simulink model "ElectricalThermalSystem"  (R2026b)
settings: Solver=VariableStepAuto
undefined symbols (not defined in the file): CtrlThrBattTrgTemp, CtrlThrCabTrgTemp, CtrlThrDCDCTrgTemp, CtrlThrEMTrgTemp, CtrlThrIceTrgTemp, CtrlThrMinSpd, CtrlThrTmDelay, EnvAirTemp, PlntBattCp, PlntBattMass, PlntDCDCMass, PlntEMCp, PlntEMMass, PlntEngFuelLhv, PlntThrAirCp, PlntThrAirCpBpt, PlntThrBattTau, PlntThrCabHtc, PlntThrCabNPass, PlntThrCabTau, PlntThrCabVolume, PlntThrCoolCp, PlntThrCoolCpBpt, PlntThrCOPc, PlntThrCOPe, PlntThrDCDCTau, PlntThrDoorsArea, PlntThrDoorsK, PlntThrDoorsTk, PlntThrEMTau, PlntThrGlassArea, PlntThrGlassK, PlntThrGlassTk, PlntThrICETau, PlntThrRoofArea, PlntThrRoofK, PlntThrRoofTk
libraries: simulink x2, autolibutils x1
settings Model: ModifiedByFormat=The MathWorks, Inc.  Creator=The MathWorks, Inc.  LastModifiedBy=The MathWorks, Inc.
settings RTWCC: LargeConstantGeneration=WriteOnlyDNNConstantsToDataFiles

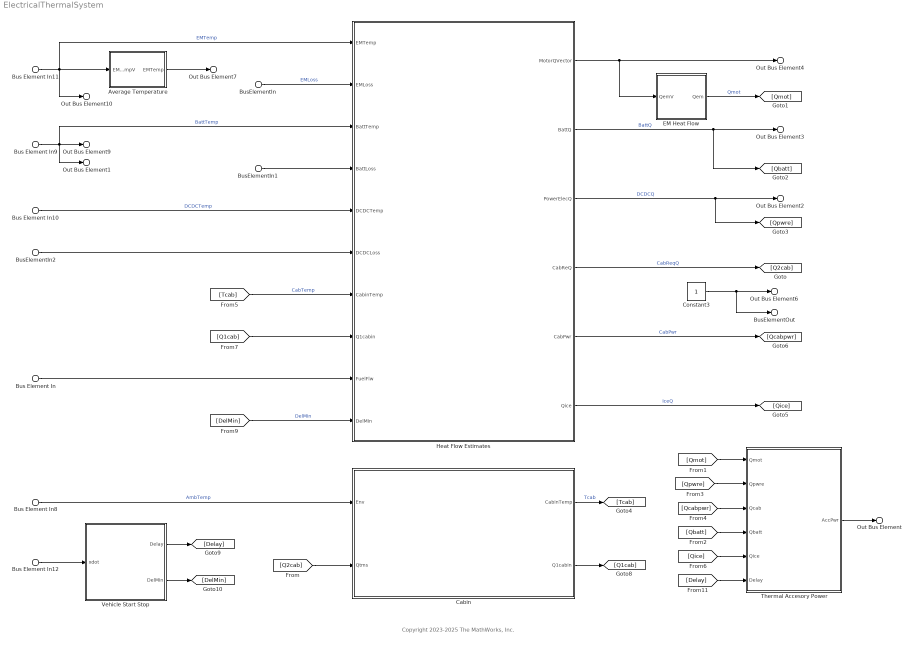
== system ElectricalThermalSystem ==
  note: Copyright 2023-2025 The MathWorks, Inc.
  Bus Element In8 : Inport  PortName=Env  Element=AmbTemp
  Bus Element In9 : Inport  Port=2  PortName=Battery  Element=BattInfo.BattTemp
  BusElementIn1 : Inport  Port=2  PortName=Battery  Element=BattInfo.BattPwrLoss
  Bus Element In10 : Inport  Port=3  PortName=PwrElec  Element=PwrETemp
  BusElementIn2 : Inport  Port=3  PortName=PwrElec  Element=PwrELoss
  Bus Element In11 : Inport  Port=4  PortName=ElecMachine  Element=EMTemp
  BusElementIn : Inport  Port=4  PortName=ElecMachine  Element=EMPwrLoss
  Bus Element In12 : Inport  Port=5  PortName=VehBody  Element=BdyFrm.Cg.Vel.xdot
  Bus Element In : Inport  Port=6  PortName=Eng  Element=FuelFlw
  Average Temperature : Subsystem
  Cabin : Subsystem
  Constant3 : Constant  SampleTime=-1
  EM Heat Flow : Subsystem  Variant=on
  Heat Flow Estimates : Subsystem
  Thermal Accesory Power : Subsystem  mask{COPe=PlntThrCOPe, COPc=PlntThrCOPc}
      mask prompts: COPe "E-Cab coefficient of performance, COPe []"; COPc "ICE coefficient of performance, COPc []"
      mask help: Estimates the power required to operate the thermal management. E-Cab coefficient of performance is the ratio of the absolute value of heat transferred to or from all electric subsystems and cabin over the power required. ICE coefficient of performance is the ratio of heat transferred to cool the internal combustion engine over the power required (applies only to HEV).
  Vehicle Start Stop : Subsystem
  Out Bus Element7 : Outport  PortName=Thermal  Element=EMCoolTempOut
  Out Bus Element9 : Outport  PortName=Thermal  Element=BattTemp
  Out Bus Element10 : Outport  PortName=Thermal  Element=MotorTemp
  Out Bus Element6 : Outport  PortName=Thermal  Element=CondPress
  Out Bus Element : Outport  PortName=Thermal  Element=EAccPwr
  Out Bus Element1 : Outport  PortName=Thermal  Element=BattCoolTemp
  Out Bus Element3 : Outport  PortName=Thermal  Element=Qbatt
  Out Bus Element2 : Outport  PortName=Thermal  Element=Qpwre
  Out Bus Element4 : Outport  PortName=Thermal  Element=Qem
  BusElementOut : Outport  PortName=Thermal  Element=EvapPress
  wires:
  Bus Element In/1 -> Heat Flow Estimates/9(FuelFlw)
  [Delay] -> Thermal Accesory Power/6(Delay)
  Bus Element In12/1 -> Vehicle Start Stop/1(xdot)
  Vehicle Start Stop/2(DelMin) -> [DelMin]
  Vehicle Start Stop/1(Delay) -> [Delay]
  Heat Flow Estimates/5(CabPwr) -> [Qcabpwr]  "CabPwr"
  Heat Flow Estimates/6(Qice) -> [Qice]  "IceQ"
  [Tcab] -> Heat Flow Estimates/7(CabinTemp)  "CabTemp"
  Cabin/1(CabinTemp) -> [Tcab]  "Tcab"
  Thermal Accesory Power/1(AccPwr) -> Out Bus Element/1
  [Qbatt] -> Thermal Accesory Power/4(Qbatt)
  [Qcabpwr] -> Thermal Accesory Power/3(Qcab)
  [Qpwre] -> Thermal Accesory Power/2(Qpwre)
  [Qmot] -> Thermal Accesory Power/1(Qmot)
  Bus Element In10/1 -> Heat Flow Estimates/5(DCDCTemp)  "DCDCTemp"
  Heat Flow Estimates/2(BattQ) -> [Qbatt], Out Bus Element3/1  "BattQ"
  Heat Flow Estimates/1(MotorQVector) -> Out Bus Element4/1, EM Heat Flow/1(QemV)
  EM Heat Flow/1(Qem) -> [Qmot]  "Qmot"
  Bus Element In8/1 -> Cabin/1(Env)  "AmbTemp"
  Constant3/1 -> Out Bus Element6/1, BusElementOut/1
  [Q2cab] -> Cabin/2(Qtms)
  Bus Element In9/1 -> Heat Flow Estimates/3(BattTemp), Out Bus Element1/1, Out Bus Element9/1  "BattTemp"
  [Qice] -> Thermal Accesory Power/5(Qice)
  Heat Flow Estimates/4(CabReQ) -> [Q2cab]  "CabReqQ"
  BusElementIn/1 -> Heat Flow Estimates/2(EMLoss)  "EMLoss"
  BusElementIn1/1 -> Heat Flow Estimates/4(BattLoss)
  BusElementIn2/1 -> Heat Flow Estimates/6(DCDCLoss)
  Cabin/2(Q1cabin) -> [Q1cab]
  [Q1cab] -> Heat Flow Estimates/8(Q1cabin)
  Heat Flow Estimates/3(PowerElecQ) -> Out Bus Element2/1, [Qpwre]  "DCDCQ"
  Bus Element In11/1 -> Heat Flow Estimates/1(EMTemp), Out Bus Element10/1, Average Temperature/1(EMTempV)  "EMTemp"
  Average Temperature/1(EMTemp) -> Out Bus Element7/1
  [DelMin] -> Heat Flow Estimates/10(DelMin)  "DelMin"

== system ElectricalThermalSystem/Average Temperature ==
  EMTempV : Inport
  Divide3 : Product  Inputs=*/
  Sum of Elements : Sum  Inputs=+
  Width : Width
  EMTemp : Outport
  wires:
  Sum of Elements/1 -> Divide3/1
  Divide3/1 -> EMTemp/1
  Width/1 -> Divide3/2
  EMTempV/1 -> Sum of Elements/1, Width/1

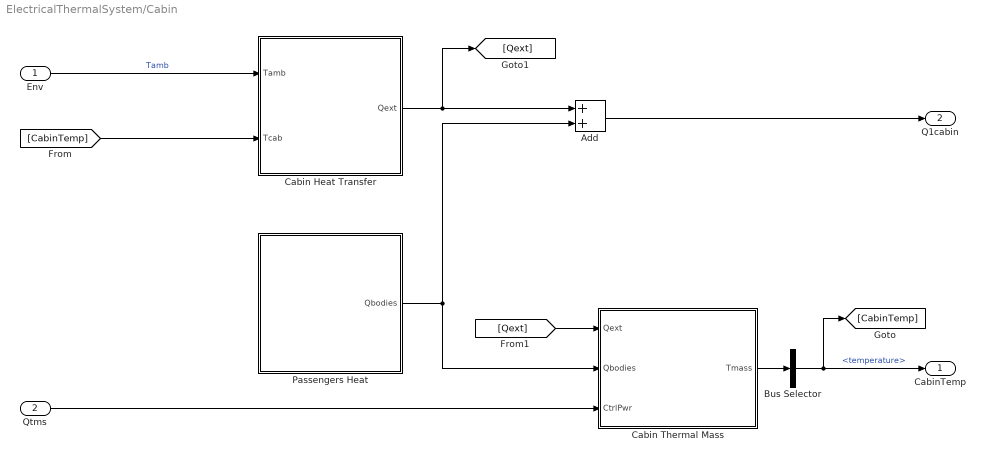
== system ElectricalThermalSystem/Cabin ==
  Env : Inport
  Qtms : Inport  Port=2
  Add : Sum
  Bus Selector : BusSelector  OutputSignals=temperature
  Cabin Heat Transfer : Subsystem
  Cabin Thermal Mass : Subsystem  mask{Vol=PlntThrCabVolume, HeatCp=PlntThrAirCp, HeatBrkPts=PlntThrAirCpBpt}
      mask prompts: Vol "Volume, Vol [m^3]"; HeatCp "Specific heat capacity, HeatCp [J/(kg*K)]"; HeatBrkPts "Specific heat capacity brk pts, HeatBrkPts [K]"
      settings: LibrarySourceBlock=autolibsharedcommon/Thermal Mass
      mask TypeOptions Vol: Volume/Value
      mask TypeOptions HeatCp: HeatCp/Value
      mask TypeOptions HeatBrkPts: Specific Heat/BreakpointsForDimension1
      mask DialogControl DescTextVar Prompt: For an air volume, estimates the instantaneous temperature given the heat transfer balance
  Passengers Heat : Subsystem
  CabinTemp : Outport
  Q1cabin : Outport  Port=2
  wires:
  Add/1 -> Q1cabin/1
  [Qext] -> Cabin Thermal Mass/1(Qext)
  Env/1 -> Cabin Heat Transfer/1(Tamb)  "Tamb"
  [CabinTemp] -> Cabin Heat Transfer/2(Tcab)
  Passengers Heat/1(Qbodies) -> Cabin Thermal Mass/2(Qbodies), Add/2
  Cabin Heat Transfer/1(Qext) -> Add/1, [Qext]
  Qtms/1 -> Cabin Thermal Mass/3(CtrlPwr)
  Cabin Thermal Mass/1(Tmass) -> Bus Selector/1
  Bus Selector/1 -> [CabinTemp], CabinTemp/1  "<temperature>"

== system ElectricalThermalSystem/EM Heat Flow ==
  QemV : Inport
  FourEM : Subsystem  VariantControl=PlntEMNum == 4
  OneEM : Subsystem  VariantControl=PlntEMNum == 1
  ThreeEM : Subsystem  VariantControl=PlntEMNum == 3
  TwoEM : Subsystem  VariantControl=PlntEMNum == 2
  Qem : Outport

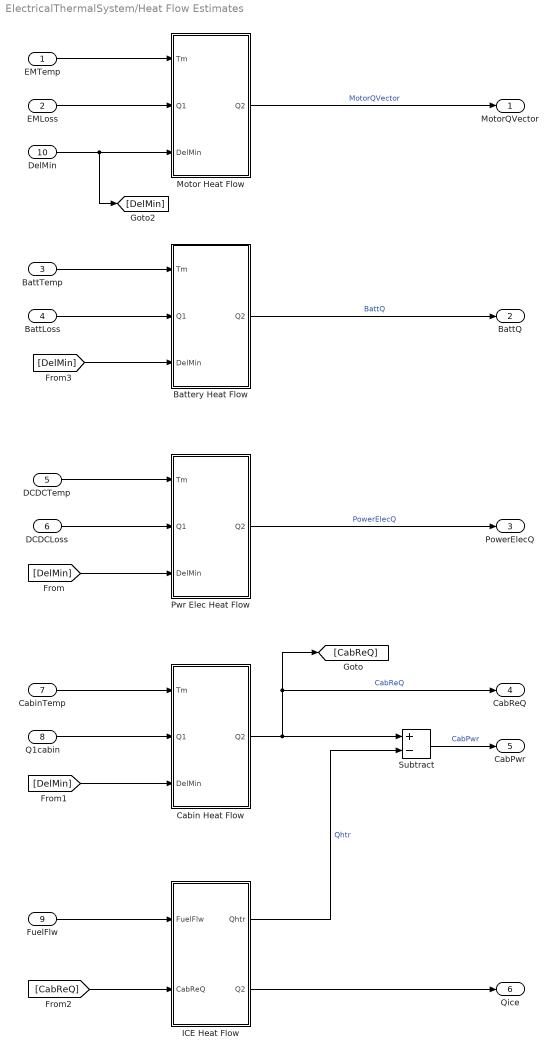
== system ElectricalThermalSystem/Heat Flow Estimates ==
  EMTemp : Inport
  EMLoss : Inport  Port=2
  BattTemp : Inport  Port=3
  BattLoss : Inport  Port=4
  DCDCTemp : Inport  Port=5
  DCDCLoss : Inport  Port=6
  CabinTemp : Inport  Port=7
  Q1cabin : Inport  Port=8
  FuelFlw : Inport  Port=9
  DelMin : Inport  Port=10
  Battery Heat Flow : Subsystem  mask{TrgT=CtrlThrBattTrgTemp, Cp=PlntBattCp, Mass=PlntBattMass, Tau=PlntThrBattTau}
      mask prompts: TrgT "Battery target temperature, TrgT [K}"; Cp "Heat capacity, Cp [J/(kg*K)]"; Mass "Mass, Mass [kg]"; Tau "Time constant, Tau [s]"
      mask TypeOptions TrgT: Constant1/Value
  Cabin Heat Flow : Subsystem  mask{TrgT=CtrlThrCabTrgTemp, Vol=PlntThrCabVolume, Cp=PlntThrAirCp, CpBpt=PlntThrAirCpBpt, Tau=PlntThrCabTau}
      mask prompts: TrgT "Cabin target temperature, TrgT [K}"; Vol "Cabin volume, Vol [m^3]"; Cp "Air heat capacity, Cp [J/(kg*K)]"; CpBpt "Heat capacity breakpoints, CpBpt [K]"; Tau "Time constant, Tau [s]"
      mask TypeOptions TrgT: Constant1/Value
      mask TypeOptions Vol: CabinVolume/Value
      mask TypeOptions Cp: Specific Heat/Table
      mask TypeOptions CpBpt: Specific Heat/BreakpointsForDimension1
  ICE Heat Flow : Subsystem  Variant=on  VariantControlMode=label  LabelModeActiveChoice=NoICE
  Motor Heat Flow : Subsystem  mask{TrgT=CtrlThrEMTrgTemp, Cp=PlntEMCp, Mass=PlntEMMass, Tau=PlntThrEMTau}
      mask prompts: TrgT "Motor target temperature, TrgT [K]"; Cp "Heat capacity, Cp [J/(kg*K)]"; Mass "Mass, Mass [kg]"; Tau "Time constant, Tau [s]"
      mask TypeOptions TrgT: Constant1/Value
  Pwr Elec Heat Flow : Subsystem  mask{TrgT=CtrlThrDCDCTrgTemp, Cp=PlntEMCp, Mass=PlntDCDCMass, Tau=PlntThrDCDCTau}
      mask prompts: TrgT "DCDC Converter target temperature, TrgT [K}"; Cp "Heat capacity, Cp [J/(kg*K)]"; Mass "Mass, Mass [kg]"; Tau "Time constant, Tau [s]"
      mask TypeOptions TrgT: Constant1/Value
  Subtract : Sum  Inputs=+-
  MotorQVector : Outport
  BattQ : Outport  Port=2
  PowerElecQ : Outport  Port=3
  CabReQ : Outport  Port=4
  CabPwr : Outport  Port=5
  Qice : Outport  Port=6
  wires:
  ICE Heat Flow/2(Q2) -> Qice/1
  Q1cabin/1 -> Cabin Heat Flow/2(Q1)
  DCDCLoss/1 -> Pwr Elec Heat Flow/2(Q1)
  BattLoss/1 -> Battery Heat Flow/2(Q1)
  EMLoss/1 -> Motor Heat Flow/2(Q1)
  FuelFlw/1 -> ICE Heat Flow/1(FuelFlw)
  CabinTemp/1 -> Cabin Heat Flow/1(Tm)
  DCDCTemp/1 -> Pwr Elec Heat Flow/1(Tm)
  BattTemp/1 -> Battery Heat Flow/1(Tm)
  EMTemp/1 -> Motor Heat Flow/1(Tm)
  Battery Heat Flow/1(Q2) -> BattQ/1  "BattQ"
  Motor Heat Flow/1(Q2) -> MotorQVector/1  "MotorQVector"
  Pwr Elec Heat Flow/1(Q2) -> PowerElecQ/1  "PowerElecQ"
  Cabin Heat Flow/1(Q2) -> [CabReQ], CabReQ/1, Subtract/1  "CabReQ"
  [CabReQ] -> ICE Heat Flow/2(CabReQ)
  ICE Heat Flow/1(Qhtr) -> Subtract/2  "Qhtr"
  Subtract/1 -> CabPwr/1  "CabPwr"
  [DelMin] -> Cabin Heat Flow/3(DelMin)
  [DelMin] -> Pwr Elec Heat Flow/3(DelMin)
  DelMin/1 -> [DelMin], Motor Heat Flow/3(DelMin)
  [DelMin] -> Battery Heat Flow/3(DelMin)

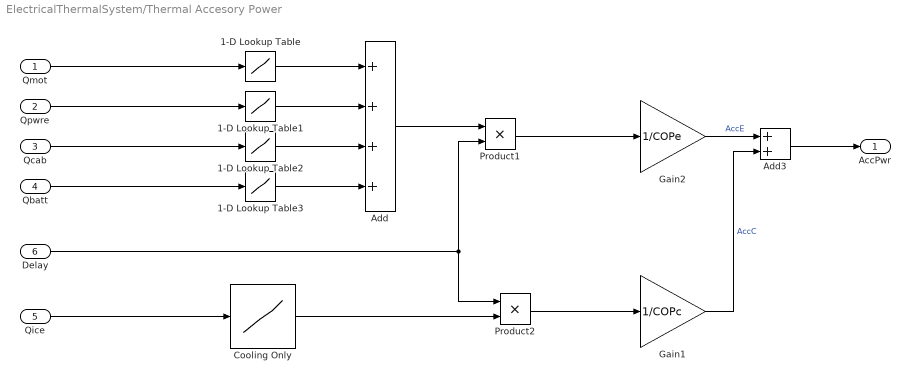
== system ElectricalThermalSystem/Thermal Accesory Power ==
  Qmot : Inport
  Qpwre : Inport  Port=2
  Qcab : Inport  Port=3
  Qbatt : Inport  Port=4
  Qice : Inport  Port=5
  Delay : Inport  Port=6
  1-D Lookup Table{,1..3} (4 alike) : Lookup_n-D  NumberOfTableDimensions=1  BreakpointsForDimension1=[-1 0 1]  Table=[1 0 1]  InternalRulePriority=Speed  RndMeth=Simplest
  Add : Sum  Inputs=++++
  Add3 : Sum
  Cooling Only : Lookup_n-D  NumberOfTableDimensions=1  BreakpointsForDimension1=[-1 0 1]  Table=[1 0 0]  InternalRulePriority=Speed  RndMeth=Simplest
  Gain1 : Gain  Gain=1/COPc
  Gain2 : Gain  Gain=1/COPe
  Product1 : Product
  Product2 : Product
  AccPwr : Outport
  wires:
  Add3/1 -> AccPwr/1
  Gain1/1 -> Add3/2  "AccC"
  Gain2/1 -> Add3/1  "AccE"
  Qice/1 -> Cooling Only/1
  Qpwre/1 -> 1-D Lookup Table1/1
  Qmot/1 -> 1-D Lookup Table/1
  Qcab/1 -> 1-D Lookup Table2/1
  Qbatt/1 -> 1-D Lookup Table3/1
  Add/1 -> Product1/1
  Product2/1 -> Gain1/1
  Delay/1 -> Product1/2, Product2/1
  Cooling Only/1 -> Product2/2
  1-D Lookup Table2/1 -> Add/3
  1-D Lookup Table3/1 -> Add/4
  1-D Lookup Table/1 -> Add/1
  1-D Lookup Table1/1 -> Add/2
  Product1/1 -> Gain2/1

== system ElectricalThermalSystem/Vehicle Start Stop ==
  xdot : Inport
  Compare To Constant : simulink/Logic and Bit Operations/Compare To Constant  relop=>=  const=CtrlThrMinSpd  OutDataTypeStr=boolean
  Delayed Stop : Subsystem
  Gain1 : Gain
  Minimum heat transfer1 : Lookup_n-D  NumberOfTableDimensions=1  BreakpointsForDimension1=[0 1]  Table=[0.1 1]  ExtrapMethod=Clip  InternalRulePriority=Speed  RndMeth=Simplest
  Delay : Outport
  DelMin : Outport  Port=2
  wires:
  xdot/1 -> Compare To Constant/1
  Delayed Stop/1(On) -> Delay/1, Gain1/1
  Compare To Constant/1 -> Delayed Stop/1(Moving)
  Minimum heat transfer1/1 -> DelMin/1
  Gain1/1 -> Minimum heat transfer1/1

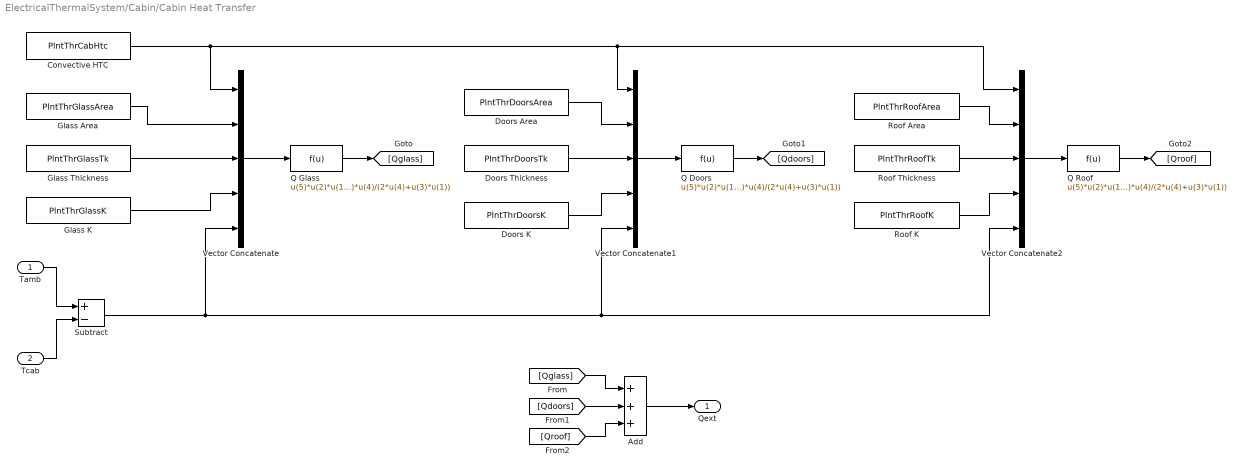
== system ElectricalThermalSystem/Cabin/Cabin Heat Transfer ==
  Tamb : Inport
  Tcab : Inport  Port=2
  Add : Sum  Inputs=+++
  Convective HTC : Constant  Value=PlntThrCabHtc  SampleTime=-1
  Doors Area : Constant  Value=PlntThrDoorsArea  SampleTime=-1
  Doors K : Constant  Value=PlntThrDoorsK  SampleTime=-1
  Doors Thickness : Constant  Value=PlntThrDoorsTk  SampleTime=-1
  Glass Area : Constant  Value=PlntThrGlassArea  SampleTime=-1
  Glass K : Constant  Value=PlntThrGlassK  SampleTime=-1
  Glass Thickness : Constant  Value=PlntThrGlassTk  SampleTime=-1
  Q Doors : Fcn  Expr=u(5)*u(2)*u(1)*u(4)/(2*u(4)+u(3)*u(1))
  Q Glass : Fcn  Expr=u(5)*u(2)*u(1)*u(4)/(2*u(4)+u(3)*u(1))
  Q Roof : Fcn  Expr=u(5)*u(2)*u(1)*u(4)/(2*u(4)+u(3)*u(1))
  Roof Area : Constant  Value=PlntThrRoofArea  SampleTime=-1
  Roof K : Constant  Value=PlntThrRoofK  SampleTime=-1
  Roof Thickness : Constant  Value=PlntThrRoofTk  SampleTime=-1
  Subtract : Sum  Inputs=+-
  Vector Concatenate : Concatenate  NumInputs=5
  Vector Concatenate1 : Concatenate  NumInputs=5
  Vector Concatenate2 : Concatenate  NumInputs=5
  Qext : Outport
  wires:
  Tamb/1 -> Subtract/1
  Tcab/1 -> Subtract/2
  Convective HTC/1 -> Vector Concatenate2/1, Vector Concatenate1/1, Vector Concatenate/1
  Subtract/1 -> Vector Concatenate2/5, Vector Concatenate1/5, Vector Concatenate/5
  Glass Thickness/1 -> Vector Concatenate/3
  Glass Area/1 -> Vector Concatenate/2
  Glass K/1 -> Vector Concatenate/4
  Doors Thickness/1 -> Vector Concatenate1/3
  Doors Area/1 -> Vector Concatenate1/2
  Doors K/1 -> Vector Concatenate1/4
  Roof Thickness/1 -> Vector Concatenate2/3
  Roof Area/1 -> Vector Concatenate2/2
  Roof K/1 -> Vector Concatenate2/4
  Vector Concatenate/1 -> Q Glass/1
  Vector Concatenate1/1 -> Q Doors/1
  Vector Concatenate2/1 -> Q Roof/1
  Q Glass/1 -> [Qglass]
  Q Doors/1 -> [Qdoors]
  Q Roof/1 -> [Qroof]
  [Qdoors] -> Add/2
  Add/1 -> Qext/1
  [Qglass] -> Add/1
  [Qroof] -> Add/3

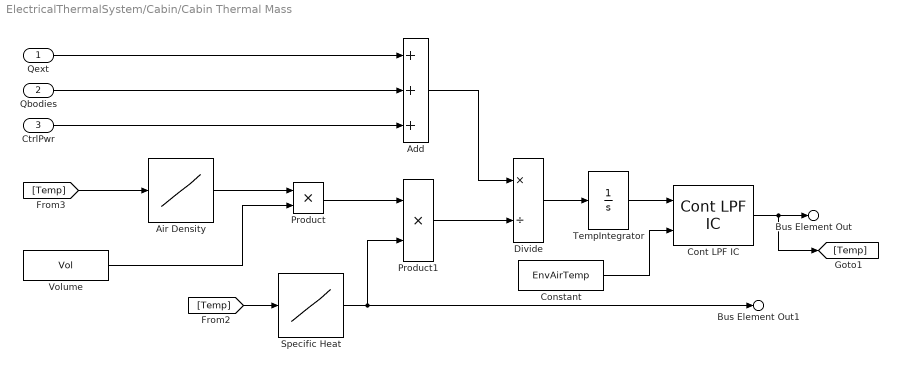
== system ElectricalThermalSystem/Cabin/Cabin Thermal Mass ==
  Qext : Inport
  Qbodies : Inport  Port=2
  CtrlPwr : Inport  Port=3
  Add : Sum  Inputs=+++
  Air Density : Lookup_n-D  NumberOfTableDimensions=1  BreakpointsForDimension1=[248.14999999999998 263.15 273.15 283.15 293.15 298.15 303.15 313.15 333.15 373.15 473.15 573.15]  Table=[1.42 1.341 1.2922 1.2466 1.204 1.18 1.16 1.1 1.025 0.916 0.723 0.596]  ExtrapMethod=Clip  InternalRulePriority=Speed  RndMeth=Simplest
  Constant : Constant  Value=EnvAirTemp
  Cont LPF IC : autolibutils/Cont LPF IC  wc=0.1/Vol  aMode=aMode  dataType=off
  Divide : Product  Inputs=*/
  Product : Product
  Product1 : Product
  Specific Heat : Lookup_n-D  NumberOfTableDimensions=1  BreakpointsForDimension1=HeatBrkPts  Table=HeatCp  ExtrapMethod=Clip  UseLastTableValue=on  InternalRulePriority=Speed  RndMeth=Simplest
  TempIntegrator : Integrator  InitialCondition=EnvAirTemp
  Volume : Constant  Value=Vol  VectorParams1D=off  SampleTime=-1
  Bus Element Out : Outport  PortName=Tmass  Element=temperature
  Bus Element Out1 : Outport  PortName=Tmass  Element=cp
  wires:
  Product1/1 -> Divide/2
  Product/1 -> Product1/1
  [Temp] -> Specific Heat/1
  Specific Heat/1 -> Bus Element Out1/1, Product1/2
  Air Density/1 -> Product/1
  Volume/1 -> Product/2
  Add/1 -> Divide/1
  Divide/1 -> TempIntegrator/1
  Qbodies/1 -> Add/2
  Qext/1 -> Add/1
  [Temp] -> Air Density/1
  CtrlPwr/1 -> Add/3
  TempIntegrator/1 -> Cont LPF IC/1
  Cont LPF IC/1 -> [Temp], Bus Element Out/1
  Constant/1 -> Cont LPF IC/2

== system ElectricalThermalSystem/Cabin/Passengers Heat ==
  Body Heat : Constant  Value=70  SampleTime=-1
  Constant : Constant  Value=PlntThrCabNPass  SampleTime=-1
  Product : Product
  Qbodies : Outport
  wires:
  Body Heat/1 -> Product/2
  Constant/1 -> Product/1
  Product/1 -> Qbodies/1

== system ElectricalThermalSystem/EM Heat Flow/FourEM ==
  QemV : Inport
  Add : Sum  Inputs=++++
  Selector : Selector  InputPortWidth=PlntEMNum  IndexOptions=Index vector (dialog)  Indices=1  OutputSizes=1  RuntimeRangeChecks=off
  Selector1 : Selector  InputPortWidth=PlntEMNum  IndexOptions=Index vector (dialog)  Indices=2  OutputSizes=1  RuntimeRangeChecks=off
  Selector2 : Selector  InputPortWidth=PlntEMNum  IndexOptions=Index vector (dialog)  Indices=3  OutputSizes=1  RuntimeRangeChecks=off
  Selector3 : Selector  InputPortWidth=PlntEMNum  IndexOptions=Index vector (dialog)  Indices=4  OutputSizes=1  RuntimeRangeChecks=off
  Qem : Outport
  wires:
  Selector3/1 -> Add/4
  Selector2/1 -> Add/3
  Add/1 -> Qem/1
  Selector1/1 -> Add/2
  Selector/1 -> Add/1
  QemV/1 -> Selector/1, Selector1/1, Selector2/1, Selector3/1

== system ElectricalThermalSystem/EM Heat Flow/OneEM ==
  QemV : Inport
  Selector : Selector  InputPortWidth=PlntEMNum  IndexOptions=Index vector (dialog)  Indices=1  OutputSizes=1  RuntimeRangeChecks=off
  Qem : Outport
  wires:
  Selector/1 -> Qem/1
  QemV/1 -> Selector/1

== system ElectricalThermalSystem/EM Heat Flow/ThreeEM ==
  QemV : Inport
  Add : Sum  Inputs=+++
  Selector : Selector  InputPortWidth=PlntEMNum  IndexOptions=Index vector (dialog)  Indices=1  OutputSizes=1  RuntimeRangeChecks=off
  Selector1 : Selector  InputPortWidth=PlntEMNum  IndexOptions=Index vector (dialog)  Indices=2  OutputSizes=1  RuntimeRangeChecks=off
  Selector2 : Selector  InputPortWidth=PlntEMNum  IndexOptions=Index vector (dialog)  Indices=3  OutputSizes=1  RuntimeRangeChecks=off
  Qem : Outport
  wires:
  Selector2/1 -> Add/3
  Add/1 -> Qem/1
  Selector1/1 -> Add/2
  Selector/1 -> Add/1
  QemV/1 -> Selector/1, Selector1/1, Selector2/1

== system ElectricalThermalSystem/EM Heat Flow/TwoEM ==
  QemV : Inport
  Add : Sum
  Selector : Selector  InputPortWidth=PlntEMNum  IndexOptions=Index vector (dialog)  Indices=1  OutputSizes=1  RuntimeRangeChecks=off
  Selector1 : Selector  InputPortWidth=PlntEMNum  IndexOptions=Index vector (dialog)  Indices=2  OutputSizes=1  RuntimeRangeChecks=off
  Qem : Outport
  wires:
  Add/1 -> Qem/1
  Selector1/1 -> Add/2
  Selector/1 -> Add/1
  QemV/1 -> Selector/1, Selector1/1

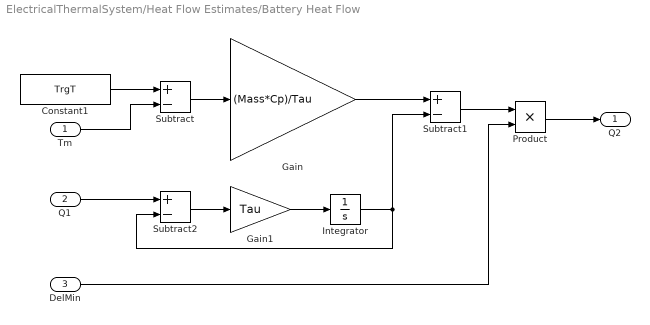
== system ElectricalThermalSystem/Heat Flow Estimates/Battery Heat Flow ==
  Tm : Inport
  Q1 : Inport  Port=2
  DelMin : Inport  Port=3
  Constant1 : Constant  Value=TrgT  SampleTime=-1
  Gain : Gain  Gain=(Mass*Cp)/Tau
  Gain1 : Gain  Gain=Tau
  Integrator : Integrator
  Product : Product
  Subtract : Sum  Inputs=+-
  Subtract1 : Sum  Inputs=+-
  Subtract2 : Sum  Inputs=+-
  Q2 : Outport
  wires:
  Subtract1/1 -> Product/1
  Subtract2/1 -> Gain1/1
  Constant1/1 -> Subtract/1
  Gain1/1 -> Integrator/1
  Gain/1 -> Subtract1/1
  Integrator/1 -> Subtract1/2, Subtract2/2
  Q1/1 -> Subtract2/1
  Tm/1 -> Subtract/2
  Subtract/1 -> Gain/1
  Product/1 -> Q2/1
  DelMin/1 -> Product/2

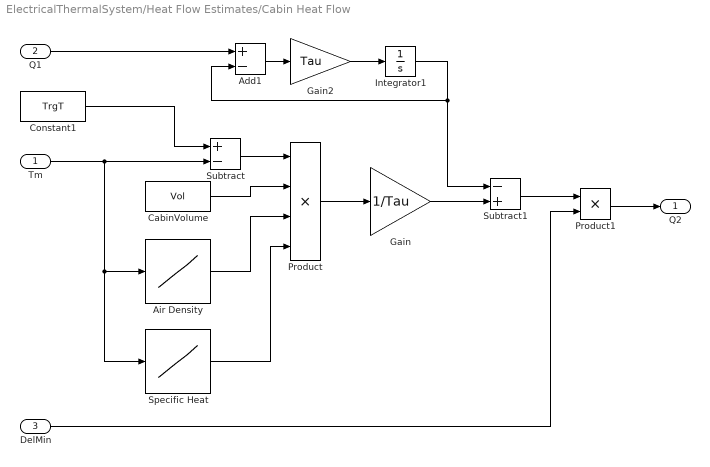
== system ElectricalThermalSystem/Heat Flow Estimates/Cabin Heat Flow ==
  Tm : Inport
  Q1 : Inport  Port=2
  DelMin : Inport  Port=3
  Add1 : Sum  Inputs=+-
  Air Density : Lookup_n-D  NumberOfTableDimensions=1  BreakpointsForDimension1=[248.14999999999998 263.15 273.15 283.15 293.15 298.15 303.15 313.15 333.15 373.15 473.15 573.15]  Table=[1.42 1.341 1.2922 1.2466 1.204 1.18 1.16 1.1 1.025 0.916 0.723 0.596]  ExtrapMethod=Clip  InternalRulePriority=Speed  RndMeth=Simplest
  CabinVolume : Constant  Value=Vol  SampleTime=-1
  Constant1 : Constant  Value=TrgT  SampleTime=-1
  Gain : Gain  Gain=1/Tau
  Gain2 : Gain  Gain=Tau
  Integrator1 : Integrator
  Product : Product  Inputs=4
  Product1 : Product
  Specific Heat : Lookup_n-D  NumberOfTableDimensions=1  BreakpointsForDimension1=CpBpt  Table=Cp  ExtrapMethod=Clip  UseLastTableValue=on  InternalRulePriority=Speed  RndMeth=Simplest
  Subtract : Sum  Inputs=+-
  Subtract1 : Sum  Inputs=-+
  Q2 : Outport
  wires:
  Integrator1/1 -> Add1/2, Subtract1/1
  Gain2/1 -> Integrator1/1
  Q1/1 -> Add1/1
  Add1/1 -> Gain2/1
  Gain/1 -> Subtract1/2
  Subtract/1 -> Product/1
  Constant1/1 -> Subtract/1
  Tm/1 -> Specific Heat/1, Air Density/1, Subtract/2
  Product/1 -> Gain/1
  CabinVolume/1 -> Product/2
  Air Density/1 -> Product/3
  Specific Heat/1 -> Product/4
  Subtract1/1 -> Product1/1
  DelMin/1 -> Product1/2
  Product1/1 -> Q2/1

== system ElectricalThermalSystem/Heat Flow Estimates/ICE Heat Flow ==
  FuelFlw : Inport
  CabReQ : Inport  Port=2
  ICE : Subsystem  VariantControl=ICE  mask{TrgT=CtrlThrIceTrgTemp, Tau=PlntThrICETau}
      mask prompts: TrgT "Engine coolant target temperature, TrgT [K}"; Tau "Time constant, Tau [s]"
      mask help: Estimates the heat flow necessary to cool the engine and the portion to heat the cabin. Both outputs are 0 when there is no ICE (i.e. EV)
      mask TypeOptions TrgT: Constant4/Value
  NoICE : Subsystem  VariantControl=NoICE
  Qhtr : Outport
  Q2 : Outport  Port=2

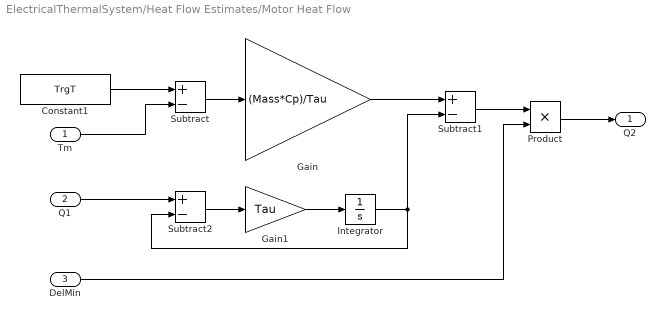
== system ElectricalThermalSystem/Heat Flow Estimates/Motor Heat Flow ==
  Tm : Inport
  Q1 : Inport  Port=2
  DelMin : Inport  Port=3
  Constant1 : Constant  Value=TrgT  SampleTime=-1
  Gain : Gain  Gain=(Mass*Cp)/Tau
  Gain1 : Gain  Gain=Tau
  Integrator : Integrator
  Product : Product
  Subtract : Sum  Inputs=+-
  Subtract1 : Sum  Inputs=+-
  Subtract2 : Sum  Inputs=+-
  Q2 : Outport
  wires:
  Q1/1 -> Subtract2/1
  Integrator/1 -> Subtract1/2, Subtract2/2
  Gain1/1 -> Integrator/1
  Subtract2/1 -> Gain1/1
  Gain/1 -> Subtract1/1
  Subtract/1 -> Gain/1
  Constant1/1 -> Subtract/1
  Tm/1 -> Subtract/2
  Subtract1/1 -> Product/1
  Product/1 -> Q2/1
  DelMin/1 -> Product/2

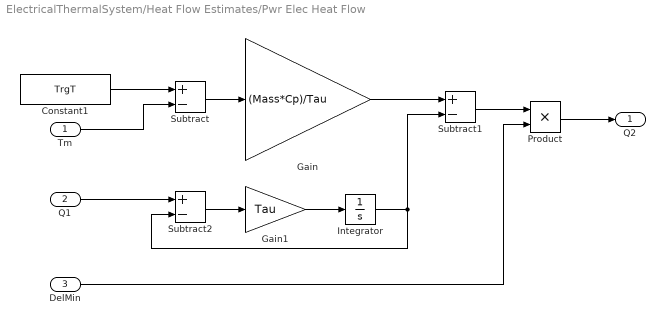
== system ElectricalThermalSystem/Heat Flow Estimates/Pwr Elec Heat Flow ==
  Tm : Inport
  Q1 : Inport  Port=2
  DelMin : Inport  Port=3
  Constant1 : Constant  Value=TrgT  SampleTime=-1
  Gain : Gain  Gain=(Mass*Cp)/Tau
  Gain1 : Gain  Gain=Tau
  Integrator : Integrator
  Product : Product
  Subtract : Sum  Inputs=+-
  Subtract1 : Sum  Inputs=+-
  Subtract2 : Sum  Inputs=+-
  Q2 : Outport
  wires:
  Subtract1/1 -> Product/1
  Subtract2/1 -> Gain1/1
  Constant1/1 -> Subtract/1
  Gain1/1 -> Integrator/1
  Gain/1 -> Subtract1/1
  Integrator/1 -> Subtract1/2, Subtract2/2
  Q1/1 -> Subtract2/1
  Tm/1 -> Subtract/2
  Subtract/1 -> Gain/1
  Product/1 -> Q2/1
  DelMin/1 -> Product/2

== system ElectricalThermalSystem/Vehicle Start Stop/Delayed Stop ==
  Moving : Inport
  Add : Sum
  Compare To Constant1 : simulink/Logic and Bit Operations/Compare To Constant  relop=>  const=CtrlThrTmDelay  OutDataTypeStr=boolean
  Constant : Constant  Value=0  SampleTime=-1
  Constant1 : Constant  Value=0.01  SampleTime=-1
  NOT1 : Logic  Operator=NOT  IconShape=distinctive  AllPortsSameDT=off  OutDataTypeStr=boolean
  Step : Step  Time=55  SampleTime=0
  Switch : Switch  Criteria=u2 > Threshold  Threshold=0.5  SaturateOnIntegerOverflow=off  InputSameDT=off
  Switch1 : Switch  Criteria=u2 > Threshold  Threshold=0.5  SaturateOnIntegerOverflow=off  InputSameDT=off
  Unit Delay : UnitDelay  SampleTime=-1
  On : Outport
  wires:
  Constant1/1 -> Add/1
  Add/1 -> Switch/3
  Switch/1 -> Compare To Constant1/1, Unit Delay/1
  Constant/1 -> Switch/1
  Moving/1 -> Switch1/3, Switch/2
  Unit Delay/1 -> Add/2
  Compare To Constant1/1 -> NOT1/1
  Step/1 -> Switch1/2
  NOT1/1 -> Switch1/1
  Switch1/1 -> On/1

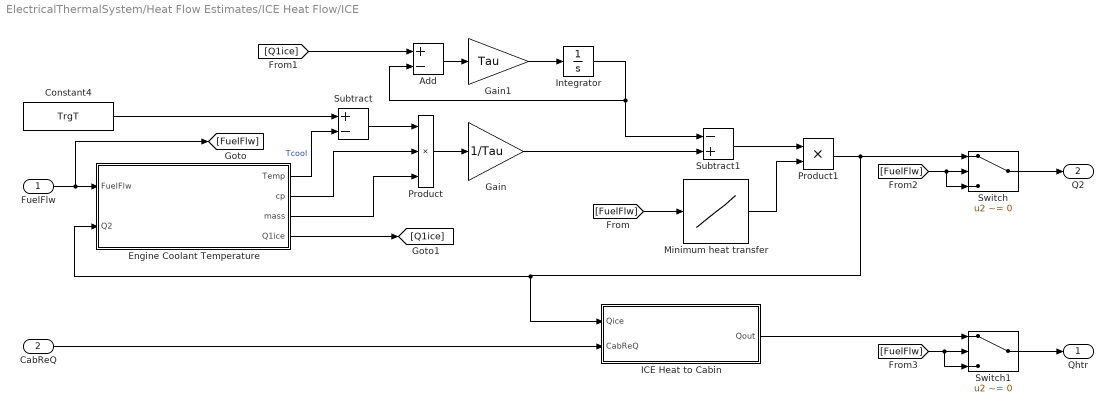
== system ElectricalThermalSystem/Heat Flow Estimates/ICE Heat Flow/ICE ==
  FuelFlw : Inport
  CabReQ : Inport  Port=2
  Add : Sum  Inputs=+-
  Constant4 : Constant  Value=TrgT  SampleTime=-1
  Engine Coolant Temperature : Subsystem
  Gain : Gain  Gain=1/Tau
  Gain1 : Gain  Gain=Tau
  ICE Heat to Cabin : Subsystem
  Integrator : Integrator
  Minimum heat transfer : Lookup_n-D  NumberOfTableDimensions=1  BreakpointsForDimension1=[0.001 0.0011]  Table=[0.1 1]  ExtrapMethod=Clip  InternalRulePriority=Speed  RndMeth=Simplest
  Product : Product  Inputs=3
  Product1 : Product
  Subtract : Sum  Inputs=+-
  Subtract1 : Sum  Inputs=-+
  Switch : Switch  Criteria=u2 ~= 0  SaturateOnIntegerOverflow=off  InputSameDT=off
  Switch1 : Switch  Criteria=u2 ~= 0  SaturateOnIntegerOverflow=off  InputSameDT=off
  Qhtr : Outport
  Q2 : Outport  Port=2
  wires:
  Integrator/1 -> Add/2, Subtract1/1
  Gain1/1 -> Integrator/1
  [Q1ice] -> Add/1
  Add/1 -> Gain1/1
  Engine Coolant Temperature/4(Q1ice) -> [Q1ice]
  Gain/1 -> Subtract1/2
  Constant4/1 -> Subtract/1
  FuelFlw/1 -> [FuelFlw], Engine Coolant Temperature/1(FuelFlw)
  CabReQ/1 -> ICE Heat to Cabin/2(CabReQ)
  Engine Coolant Temperature/1(Temp) -> Subtract/2  "Tcool"
  Subtract/1 -> Product/1
  Engine Coolant Temperature/2(cp) -> Product/2
  Engine Coolant Temperature/3(mass) -> Product/3
  Product/1 -> Gain/1
  [FuelFlw] -> Minimum heat transfer/1
  Subtract1/1 -> Product1/1
  Minimum heat transfer/1 -> Product1/2
  Product1/1 -> Switch/1, Engine Coolant Temperature/2(Q2), ICE Heat to Cabin/1(Qice)
  Switch/1 -> Q2/1
  [FuelFlw] -> Switch/3, Switch/2
  ICE Heat to Cabin/1(Qout) -> Switch1/1
  [FuelFlw] -> Switch1/3, Switch1/2
  Switch1/1 -> Qhtr/1

== system ElectricalThermalSystem/Heat Flow Estimates/ICE Heat Flow/NoICE ==
  Constant : Constant  Value=0  SampleTime=-1
  Qhtr : Outport
  Q2 : Outport  Port=2
  wires:
  Constant/1 -> Q2/1, Qhtr/1

== system ElectricalThermalSystem/Heat Flow Estimates/ICE Heat Flow/ICE/Engine Coolant Temperature ==
  FuelFlw : Inport
  Q2 : Inport  Port=2
  Bus Selector3 : BusSelector  OutputSignals=temperature,cp,mass
  Constant5 : Constant  Value=PlntEngFuelLhv  SampleTime=-1
  Gain : Gain  Gain=0.33
  Product3 : Product
  Thermal Mass : Subsystem  mask{vol=0.005, Rho=997, HeatCp=PlntThrCoolCp, HeatBrkPts=PlntThrCoolCpBpt, Tinit=EnvAirTemp}
      mask prompts: vol "Volume, vol [m^3]"; Rho "Density, Rho [kg/m^3]"; HeatCp "Specific heat capacity, HeatCp [J/(kg*K)]"; HeatBrkPts "Specific heat capacity brk pts, HeatBrkPts [K]"; Tinit "Temperature initial condition, Tinit [K]"
      mask help: For a liquid mass, estimates the instantaneous temperature given the heat transfer balance: Q1 + Q2
      mask TypeOptions vol: Volume/Value
      mask TypeOptions Rho: Rho/Value
      mask TypeOptions HeatCp: HeatCp/Value
      mask TypeOptions HeatBrkPts: Specific Heat/BreakpointsForDimension1
      mask TypeOptions Tinit: TempIntegrator/InitialCondition
  Temp : Outport
  cp : Outport  Port=2
  mass : Outport  Port=3
  Q1ice : Outport  Port=4
  wires:
  Thermal Mass/1(Tmass) -> Bus Selector3/1
  Q2/1 -> Thermal Mass/2(Q2)
  Constant5/1 -> Product3/1
  Gain/1 -> Q1ice/1, Thermal Mass/1(Q1)  "Qgas"
  Product3/1 -> Gain/1
  FuelFlw/1 -> Product3/2
  Bus Selector3/1 -> Temp/1  "<temperature>"
  Bus Selector3/2 -> cp/1  "<cp>"
  Bus Selector3/3 -> mass/1  "<mass>"

== system ElectricalThermalSystem/Heat Flow Estimates/ICE Heat Flow/ICE/ICE Heat to Cabin ==
  Qice : Inport
  CabReQ : Inport  Port=2
  Cabin Heater : Lookup_n-D  NumberOfTableDimensions=1  BreakpointsForDimension1=[-10000 0]  Table=[10000 0]  ExtrapMethod=Clip  InternalRulePriority=Speed  RndMeth=Simplest
  Gain : Gain  Gain=0.95
  Max : MinMax  Inputs=2
  Positive One : Lookup_n-D  NumberOfTableDimensions=1  BreakpointsForDimension1=[0 0.000001]  Table=[0 1]  ExtrapMethod=Clip  InternalRulePriority=Speed  RndMeth=Simplest
  Product : Product
  Qout : Outport
  wires:
  Qice/1 -> Cabin Heater/1
  CabReQ/1 -> Positive One/1, Max/1
  Product/1 -> Qout/1
  Positive One/1 -> Product/1
  Max/1 -> Gain/1
  Gain/1 -> Product/2
  Cabin Heater/1 -> Max/2

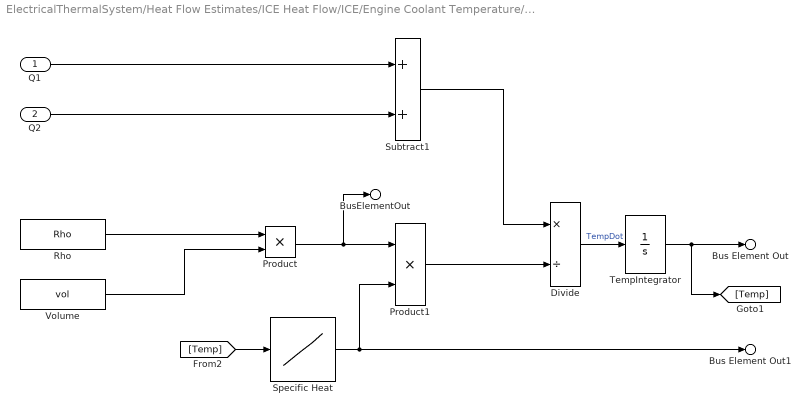
== system ElectricalThermalSystem/Heat Flow Estimates/ICE Heat Flow/ICE/Engine Coolant Temperature/Thermal Mass ==
  Q1 : Inport
  Q2 : Inport  Port=2
  Divide : Product  Inputs=*/
  Product : Product
  Product1 : Product
  Rho : Constant  Value=Rho  SampleTime=-1
  Specific Heat : Lookup_n-D  NumberOfTableDimensions=1  BreakpointsForDimension1=HeatBrkPts  Table=HeatCp  ExtrapMethod=Clip  UseLastTableValue=on  InternalRulePriority=Speed  RndMeth=Simplest
  Subtract1 : Sum
  TempIntegrator : Integrator  InitialCondition=Tinit
  Volume : Constant  Value=vol  VectorParams1D=off  SampleTime=-1
  Bus Element Out : Outport  PortName=Tmass  Element=temperature
  Bus Element Out1 : Outport  PortName=Tmass  Element=cp
  BusElementOut : Outport  PortName=Tmass  Element=mass
  wires:
  Product1/1 -> Divide/2
  Product/1 -> BusElementOut/1, Product1/1
  [Temp] -> Specific Heat/1
  Specific Heat/1 -> Bus Element Out1/1, Product1/2
  Rho/1 -> Product/1
  Volume/1 -> Product/2
  Subtract1/1 -> Divide/1
  TempIntegrator/1 -> [Temp], Bus Element Out/1
  Divide/1 -> TempIntegrator/1  "TempDot"
  Q2/1 -> Subtract1/2
  Q1/1 -> Subtract1/1
